simulink model "Buck"  (Simulink 7.9)
settings: Solver=ode23tb  SolverMode=SingleTasking  StartTime=0.0  StopTime=0.02  MaxStep=5e-6  RelTol=1e-3
libraries: powerlib x8
settings Model: Creator=patrice  LastModifiedBy=lanyi  ExtModeTrigMode=oneshot  ExtModeArmWhenConnect=off  ExtModeAutoUpdateStatusClock=off
settings DataIOCC: LimitDataPoints=off  SignalLoggingName=sigsOut
settings OptimizationCC: BooleanDataType=off  InlineInvariantSignals=on  InitFltsAndDblsToZero=on
settings DebuggingCC: SaveWithParameterizedLinksMsg=none  SignalResolutionControl=TryResolveAllWithWarning  SolverPrmCheckMsg=none  MultiTaskDSMMsg=warning  MultiTaskCondExecSysMsg=none  FcnCallInpInsideContextMsg=Use local settings  StrictBusMsg=None
settings HardwareCC: TargetUnknown=on
settings RTWCC: TemplateMakefile=grt_unix.tmf  IncludeERTFirstTime=on
settings GRTTargetCC: TargetFcnLib=ansi_tfl_tmw.mat  CombineOutputUpdateFcns=off  GRTInterface=on

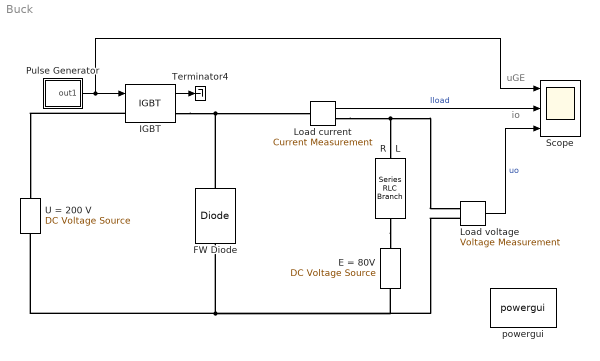
== system Buck ==
  note: io
  note: uGE
  E = 80V : powerlib/Electrical Sources/DC Voltage Source  Description=source block  Amplitude=80  Measurements=None
      settings: AttributesFormatString=\n
  FW Diode : powerlib/Power Electronics/Diode  Ron=0.01  Lon=1e-7  Vf=0.8  IC=0  UseSnubber=off  Rs=1000  Cs=0.1e-6  Measurements=off
  IGBT : powerlib/Power Electronics/IGBT  Ron=0.01  Lon=1e-6  Vf=1  Tf=1e-6  Tt=1e-6  IC=0  Rs=1000  Cs=1e-7  Measurements=on
      settings: AttributesFormatString=\n
  Load current : powerlib/Measurements/Current Measurement  Tag=PoWeRsYsTeMmEaSuReMeNt  PhasorSimulation=off  OutputType=Magnitude  PSBequivalent=0
  Load voltage : powerlib/Measurements/Voltage Measurement  Tag=PoWeRsYsTeMmEaSuReMeNt  PhasorSimulation=off  OutputType=Magnitude  PSBequivalent=0
  Pulse Generator : Subsystem  mask(Pulse Generator){period=1e-3, duty=70, amplitude=1, start=0}
      mask prompts: period "Period (secs):"; duty "Duty cycle (% of period):"; start "Start time:"
      mask help: Pulse Generator
      mask Help: Pulse generator which ensures pulse transitions are hit. Provides a vector of pulses when the height is entered as a vector.  Unmask to see how it works.
      mask Display: plot(0,0,100,100,[95,90,90,75,75,60,60,45,45,30,30,15,15,5],[25,25,75,75,25,25,75,75,25,25,75,75,25,25]);
  R   L : powerlib/Elements/Series RLC Branch  LConnTagsString=__new0  RConnTagsString=__new0  BranchType=RL  Resistance=2  Inductance=5e-03  SetiL0=off  InitialCurrent=0  Capacitance=inf  Setx0=off  InitialVoltage=0  Measurements=None
  Scope : Scope  NumInputPorts=3
      settings: TimeRange=0.01  YMin=-1~-10~-100  YMax=2~60~300  MaxDataPoints=500000
  Terminator4 : Terminator
  U = 200 V : powerlib/Electrical Sources/DC Voltage Source  Description=source block  Amplitude=200  Measurements=None
      settings: AttributesFormatString=\n
  powergui : powerlib/powergui  Priority=1  SimulationMode=Continuous  SolverType=Tustin  SampleTime=50e-6  frequency=60  SPID=off  DisableSnubberDevices=off  DisableRonSwitches=off  DisableVfSwitches=off  SwTol=0  Interpol=off  DisplayEquations=off  FunctionMessages=off  frequencyindice=0  Pbase=100e6  ErrMax=1e-4  Iterations=50  UnitsV=kV  UnitsW=MW  echomessages=off  HookPort=off  EnableUseOfTLC=off  x0status=blocks  RestoreLinks=warning  ResistiveCurrentMeasurement=off  Ylog=off  Xlog=on  ShowGrid=off  save=off  variable=ZData  ZoomFFT=off  StartTime=0.0  cycles=1  DisplayStyle=1  FreqAxis=off  MaxFrequency=1000  frequencyindicesteady=1  display=off  methode=off
  wires:
  Load current/1 -> Scope/2  "Iload"
  Load voltage/1 -> Scope/3  "uo"
  Pulse Generator/1(out1) -> IGBT/1, Scope/1
  IGBT/1 -> Terminator4/1
  connections:
  Load current/RConn1 -- Load voltage/LConn1 -- R   L/LConn1
  R   L/RConn1 -- E = 80V/RConn1
  IGBT/LConn1 -- U = 200 V/RConn1
  IGBT/RConn1 -- FW Diode/RConn1 -- Load current/LConn1
  Load voltage/LConn2 -- E = 80V/LConn1 -- U = 200 V/LConn1 -- FW Diode/LConn1

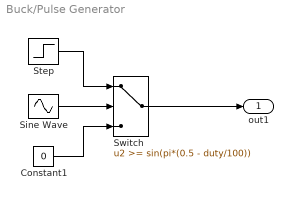
== system Buck/Pulse Generator ==
  Constant1 : Constant  Value=0
  Sine Wave : Sin  Frequency=2*pi./period  Phase=-2*pi*(start./period + duty/200 - 1/4)  SampleTime=0
  Step : Step  Time=start  After=amplitude  SampleTime=0
  Switch : Switch  Threshold=sin(pi*(0.5 - duty/100))  SaturateOnIntegerOverflow=on  InputSameDT=on
  out1 : Outport  InitialOutput=0
  wires:
  Step/1 -> Switch/1
  Constant1/1 -> Switch/3
  Switch/1 -> out1/1
  Sine Wave/1 -> Switch/2
